simulink model "ex4"  (R2020a)
settings: Solver=VariableStepAuto  StartTime=0.0  StopTime=10.0  RelTol=1e-3
values from neighbouring files (symbols this model uses):
  A = [-1 -1;6.5 0]    [Rezolvare.m]
  B = [1 1;1 0]    [Rezolvare.m]
  C = [1 0;0 1]    [Rezolvare.m]

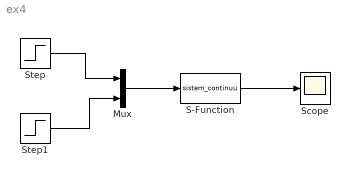
== system ex4 ==
  Mux : Mux  Inputs=2
  S-Function : S-Function  FunctionName=sistem_continuu  Parameters=A,B,C  SFunctionDeploymentMode=off  EnableBusSupport=off
  Scope : Scope
  Step : Step  SampleTime=0
  Step1 : Step  SampleTime=0
  wires:
  Step/1 -> Mux/1
  Step1/1 -> Mux/2
  Mux/1 -> S-Function/1
  S-Function/1 -> Scope/1
